simulink subsystem "Vel_Ruedas"  (R2024b)
settings: Solver=VariableStepAuto  StartTime=0.0  StopTime=10.0  RelTol=1e-3
settings Model: Creator=Chenfu  LastModifiedBy=Chenfu

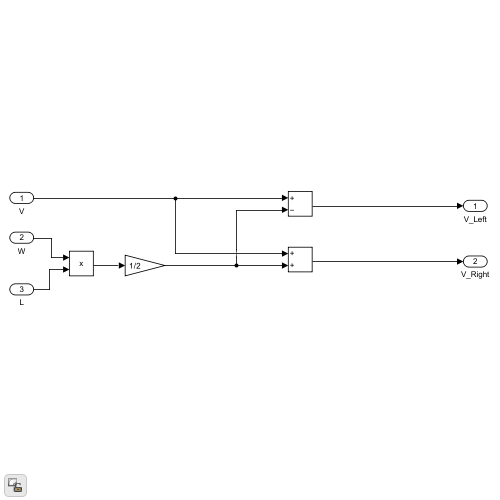
[thumbnail: Simulink's stored preview of the top-level diagram]
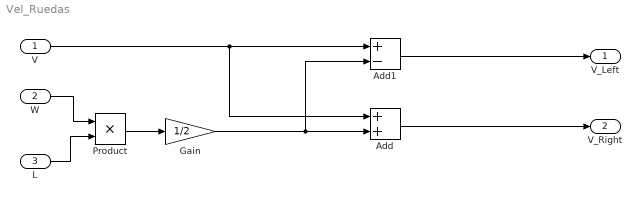
== system Vel_Ruedas ==
  V : Inport
  W : Inport  Port=2
  L : Inport  Port=3
  Add : Sum
  Add1 : Sum  Inputs=+-
  Gain : Gain  Gain=1/2
  Product : Product
  V_Left : Outport
  V_Right : Outport  Port=2
  wires:
  W/1 -> Product/1
  Product/1 -> Gain/1
  Gain/1 -> Add1/2, Add/2
  V/1 -> Add1/1, Add/1
  Add/1 -> V_Right/1
  Add1/1 -> V_Left/1
  L/1 -> Product/2
